simulink library "PhanTorque_3Dof_Library_32Bits"  (Simulink 7.6)
settings: Solver=ode45  StartTime=0.0  StopTime=10.0  RelTol=1e-3
undefined symbols (not defined in the file or in its folder): Omni_Jacobian, Omni_Jacobian_Transpose
settings Model: Creator=carlos.aldana  LastModifiedBy=carlos.aldana

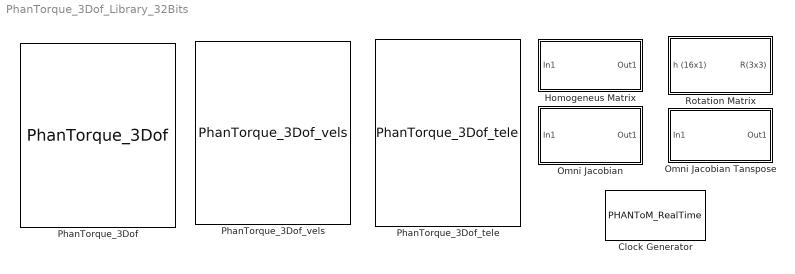
== system PhanTorque_3Dof_Library_32Bits ==
  Clock Generator : S-Function  FunctionName=PHANToM_RealTime  EnableBusSupport=off
      mask Display: text(0.1, 0.65, '\bf\fontsize{16}CPU clock', 'texmode', 'on', 'verticalAlignment', 'top', 'horizontalAlignment', 'left')
  Homogeneus Matrix : Subsystem
      mask Display:
      | text(0.5, 0.65, '\bf\fontsize{16}H', 'texmode', 'on', 'verticalAlignment', 'top', 'horizontalAlignment', 'left')
      | port_label('input', 1, 'h(16x1)')
      | port_label('output', 1, 'H(4x4)')
  Omni Jacobian : Subsystem
      mask Display:
      | text(0.4, 0.7, '\bf\fontsize{16}J', 'texmode', 'on', 'verticalAlignment', 'top', 'horizontalAlignment', 'left')
      | port_label('input', 1, 'q')
      | port_label('output', 1, 'J')
  Omni Jacobian Tanspose : Subsystem
      mask Display:
      | text(0.4, 0.7, '\bf\fontsize{16}JT', 'texmode', 'on', 'verticalAlignment', 'top', 'horizontalAlignment', 'left')
      | port_label('input', 1, 'q')
      | port_label('output', 1, 'JTrans')
  PhanTorque_3Dof : S-Function  FunctionName=PhanTorque_3Dof  Parameters=Haptic_Name  EnableBusSupport=off  mask{Haptic_Name='Default PHANToM'}
      mask prompts: Haptic_Name "Haptic Name"
      mask help:
      | Input:
      | tau--> Control Torques (3x1)
      |
      | Outputs:
      | q-->Joints Position (3x1)
      | p-->Cartesian Position (x,y,z  3x1)
      | h-->Homogeneus Transformation Matrix (vector form, 16x1)
      |
      | S-Function Parameter:
      | Haptic Name--> Name as appear on the "PHANToM Test" program.
      | ex: 'Default PHANToM'
      mask Display:
      | image(imread('omni.png'))
      | port_label('input',1,'tau');
      | port_label('output',1,'q');
      | port_label('output',2,'p');
      | port_label('output',3,'h');
  PhanTorque_3Dof_tele : S-Function  FunctionName=PhanTorque_3Dof_tele  Parameters=Haptic1_Name,Haptic2_Name  EnableBusSupport=off  mask{Haptic1_Name='Default PHANToM1', Haptic2_Name='Default PHANToM2'}
      mask prompts: Haptic1_Name "Local Haptic Name"; Haptic2_Name "Remote Haptic Name"
      mask help:
      | Input:
      | tau_l-->Local Control Torques (3x1)
      | tau_r-->Remote Control Torques (3x1)
      |
      | Outputs:
      | q_l-->Local Joints Position (3x1)
      | p_l-->Local Cartesian Position (x_l,y_l,_z_l, 3x1)
      | q_r-->Remote Joints Position (3x1)
      | p_r-->Remote Cartesian Position (x_r,y_r,z_r, 3x1)
      |
      | S-Function Parameters:
      | Haptics Names--> Names as appear on the "PHANToM Test" program.
      | ex: 'Default PHANToM'
      mask Display:
      | image(imread('2omni.png'))
      | port_label('input',1,'tau_l');
      | port_label('input',2,'tau_r');
      | port_label('output',1,'q_l');
      | port_label('output',2,'p_l');
      | port_label('output',3,'q_r');
      | port_label('output',4,'p_r');
  PhanTorque_3Dof_vels : S-Function  FunctionName=PhanTorque_3Dof_vels  Parameters=Haptic_Name  EnableBusSupport=off  mask{Haptic_Name='Default PHANToM'}
      mask prompts: Haptic_Name "Haptic Name"
      mask help:
      | Input:
      | tau--> Control Torques (3x1)
      |
      | Outputs:
      | q-->Joints Position (3x1)
      | p-->Cartesian Position (x,y,z 3x1)
      | v-->Linear Velocity (vx,vy,vz 3x1)
      | h-->Homogeneus Transformation Matrix (vector form, 16x1)
      |
      | S-Function Parameter:
      | Haptic Name--> Name as appear on the "PHANToM Test" program.
      | ex: 'Default PHANToM'
      mask Display:
      | image(imread('omni.png'))
      | port_label('input',1,'tau');
      | port_label('output',1,'q');
      | port_label('output',2,'p');
      | port_label('output',3,'v');
      | port_label('output',4,'h');
  Rotation Matrix : Subsystem
      mask Display:
      | text(0.5, 0.65, '\bf\fontsize{16}R', 'texmode', 'on', 'verticalAlignment', 'top', 'horizontalAlignment', 'left')
      | port_label('input', 1, 'h(16x1)')
      | port_label('output', 1, 'R(3x3)')

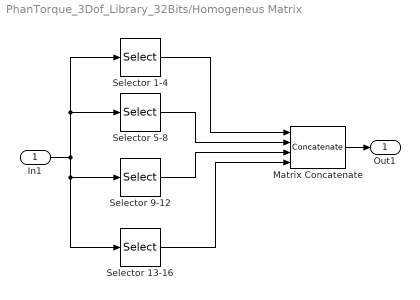
== system PhanTorque_3Dof_Library_32Bits/Homogeneus Matrix ==
  In1 : Inport
  Matrix Concatenate : Concatenate  NumInputs=4  Mode=Multidimensional array  ConcatenateDimension=2
  Selector 1-4 : Selector  InputPortWidth=16  IndexOptions=Index vector (dialog)  Indices=[1 2 3 4]  OutputSizes=1
  Selector 13-16 : Selector  InputPortWidth=16  IndexOptions=Index vector (dialog)  Indices=[13 14 15 16]  OutputSizes=1
  Selector 5-8 : Selector  InputPortWidth=16  IndexOptions=Index vector (dialog)  Indices=[5 6 7 8]  OutputSizes=1
  Selector 9-12 : Selector  InputPortWidth=16  IndexOptions=Index vector (dialog)  Indices=[9 10 11 12]  OutputSizes=1
  Out1 : Outport
  wires:
  Matrix Concatenate/1 -> Out1/1
  In1/1 -> Selector 1-4/1, Selector 5-8/1, Selector 9-12/1, Selector 13-16/1
  Selector 13-16/1 -> Matrix Concatenate/4
  Selector 9-12/1 -> Matrix Concatenate/3
  Selector 5-8/1 -> Matrix Concatenate/2
  Selector 1-4/1 -> Matrix Concatenate/1

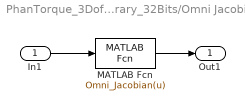
== system PhanTorque_3Dof_Library_32Bits/Omni Jacobian ==
  In1 : Inport  PortDimensions=3
  MATLAB Fcn : MATLABFcn  MATLABFcn=Omni_Jacobian(u)  OutputDimensions=[3 3]  Output1D=off
  Out1 : Outport  PortDimensions=[3 3]
  wires:
  MATLAB Fcn/1 -> Out1/1
  In1/1 -> MATLAB Fcn/1

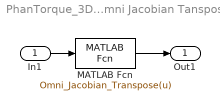
== system PhanTorque_3Dof_Library_32Bits/Omni Jacobian Tanspose ==
  In1 : Inport  PortDimensions=3
  MATLAB Fcn : MATLABFcn  MATLABFcn=Omni_Jacobian_Transpose(u)  OutputDimensions=[3 3]  Output1D=off
  Out1 : Outport  PortDimensions=[3 3]
  wires:
  In1/1 -> MATLAB Fcn/1
  MATLAB Fcn/1 -> Out1/1

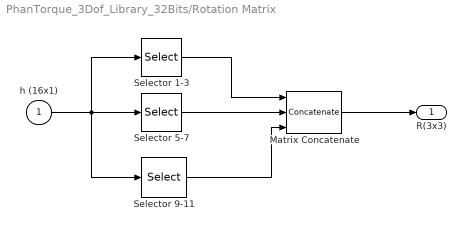
== system PhanTorque_3Dof_Library_32Bits/Rotation Matrix ==
  h (16x1) : Inport  PortDimensions=16
  Matrix Concatenate : Concatenate  NumInputs=3  Mode=Multidimensional array  ConcatenateDimension=2
  Selector 1-3 : Selector  InputPortWidth=16  IndexOptions=Index vector (dialog)  Indices=[1 2 3]  OutputSizes=1
  Selector 5-7 : Selector  InputPortWidth=16  IndexOptions=Index vector (dialog)  Indices=[5 6 7]  OutputSizes=1
  Selector 9-11 : Selector  InputPortWidth=16  IndexOptions=Index vector (dialog)  Indices=[9 10 11]  OutputSizes=1
  R(3x3) : Outport  PortDimensions=[3 3]
  wires:
  Selector 1-3/1 -> Matrix Concatenate/1
  Selector 5-7/1 -> Matrix Concatenate/2
  Selector 9-11/1 -> Matrix Concatenate/3
  Matrix Concatenate/1 -> R(3x3)/1
  h (16x1)/1 -> Selector 5-7/1, Selector 1-3/1, Selector 9-11/1
